simulink subsystem "actuator"  (R2024b)
settings: Solver=VariableStepAuto  StartTime=0.0  StopTime=10.0  RelTol=1e-3
settings Model: Creator=yagiz  LastModifiedBy=yagiz

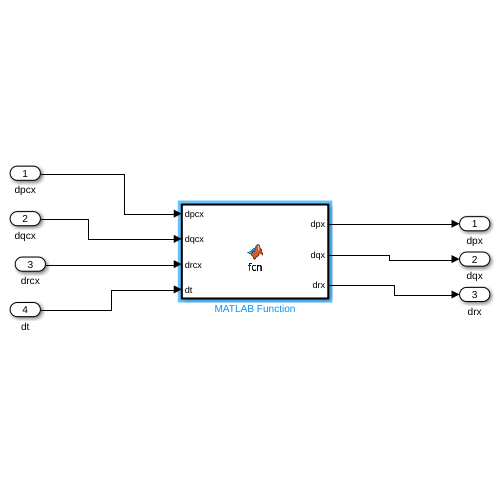
[thumbnail: Simulink's stored preview of the top-level diagram]
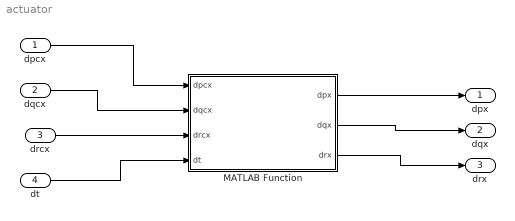
== system actuator ==
  dpcx : Inport
  dqcx : Inport  Port=2
  drcx : Inport  Port=3
  dt : Inport  Port=4
  MATLAB Function : MATLAB Function  TreatAsAtomicUnit=on
  dpx : Outport
  dqx : Outport  Port=2
  drx : Outport  Port=3
  wires:
  dpcx/1 -> MATLAB Function/1(dpcx)
  dqcx/1 -> MATLAB Function/2(dqcx)
  drcx/1 -> MATLAB Function/3(drcx)
  dt/1 -> MATLAB Function/4(dt)
  MATLAB Function/1(dpx) -> dpx/1
  MATLAB Function/2(dqx) -> dqx/1
  MATLAB Function/3(drx) -> drx/1

== matlab function actuator/MATLAB Function ==
  settings: updateMethod=DISCRETE
  data: dpcx input; dpx output; dqcx input; drcx input; dt input; dqx output; drx output
function [dpx, dqx, drx] = fcn(dpcx, dqcx, drcx, dt)

persistent del del_dot
if isempty(del)
    del     = zeros(4,1);
    del_dot = zeros(4,1);
end

dlimx  = 28.0;
ddlimx = 600.0;
wnact  = 251.0;
zetact = 0.7;
wn2    = wnact^2;

% Commands → 4 fins
delcx = [-dpcx+dqcx-drcx;
         -dpcx+dqcx+drcx;
         +dpcx+dqcx-drcx;
         +dpcx+dqcx+drcx];

% Second-order ODE
del_ddot    = wn2*(delcx - del) - 2*zetact*wnact*del_dot;

% Rate integration + limit
del_dot_new = del_dot + del_ddot * dt;
del_dot_new = max(-ddlimx, min(ddlimx, del_dot_new));

% Position integration + limit
del_new     = del + del_dot * dt;
del_new     = max(-dlimx, min(dlimx, del_new));

del     = del_new;
del_dot = del_dot_new;

% 4 fins → channels
dpx = (-del(1) - del(2) + del(3) + del(4)) / 4;
dqx = (+del(1) + del(2) + del(3) + del(4)) / 4;
drx = (-del(1) + del(2) - del(3) + del(4)) / 4;
